simulink model "L4_SIM"  (R2018a)
settings: Solver=ode1  StartTime=0.0  StopTime=60  FixedStep=GLB_FIXED_STEP_SIZE_CPV  RelTol=1e-3  EnableMultiTasking=on
undefined symbols (not defined in the file or in its folder): Cf, Chassis, Cr, CYCLE_ACC1_2A__AdaptiveCruiseCtrlMode, CYCLE_ACC1_2A__AdaptiveCruiseCtrlSetSpeed, CYCLE_CCVS1_00__CruiseCtrlSetSpeed, CYCLE_CCVS1_00__WheelBasedVehicleSpeed, CYCLE_EEC1_00__EngSpeed, CYCLE_ETC1_00__TransDrivelineEngaged, CYCLE_ETC2_00__TransActualGearRatio, CYCLE_ETC7_03__TransMode1Indicator, CYCLE_GPS_Latitude, CYCLE_GPS_Longitude, CYCLE_LFE1_00__EngFuelRate, CYCLE_Net_Engine_Percent_Torque, CYCLE_SSI2_03__PitchAngleExRange, CYCLE_TIME, CYCLE_UTM_Origin_X, CYCLE_UTM_Origin_Y, CYCLE_Vehicle_Distance, DiscIntNeverNeededParam, ENUM_J1939_PCC_STATE_T, ENUM_J1939_SWITCH_T, ENUM_STEERING_WHEEL_ANGLE_SENSOR_TYPE_T, GLB_FIXED_STEP_SIZE_CPV, GLB_TRANS_LOSS_TRQ_GEAR_STEP_MPV, GLB_TRANS_LOSS_TRQ_SPD_STEP_MPV, GLB_TRANS_LOSS_TRQ_TABLE_DATA_MPV, GLB_TRANS_LOSS_TRQ_TRQ_STEP_MPV, GLB_VEHICLE_CONFIG_ACCEL_PED_GATEWAY_APV, heading_0, Iz, L4_Controller, lf, lr, position_0, ptc_matlab_lib, STEERCTRL_10ms, SUB_ECU_L4_MABX, SUB_L4_Task_10ms, SUB_L4_Task_10ms_SUB_STEERCTRL, SUB_PLANT_Chassis, Task_10ms, Vx_0
libraries: EmE_MBD_Blockset x81, PTC_MBDS_LIB x71, simulink x38, simulink_extras x1, SUB_L4_Task_10000ms x1, SUB_L4_Task_1000ms x1, SUB_L4_Task_100ms x1, SUB_L4_Task_10ms_SUB_APTC x1, SUB_L4_Task_10ms_SUB_BRKPEDARB x1, SUB_L4_Task_10ms_SUB_FAULT_MANAGER x1, SUB_L4_Task_10ms_SUB_STATE_CONTROL x1, simulink_need_slupdate x1
(part 4 of 6)

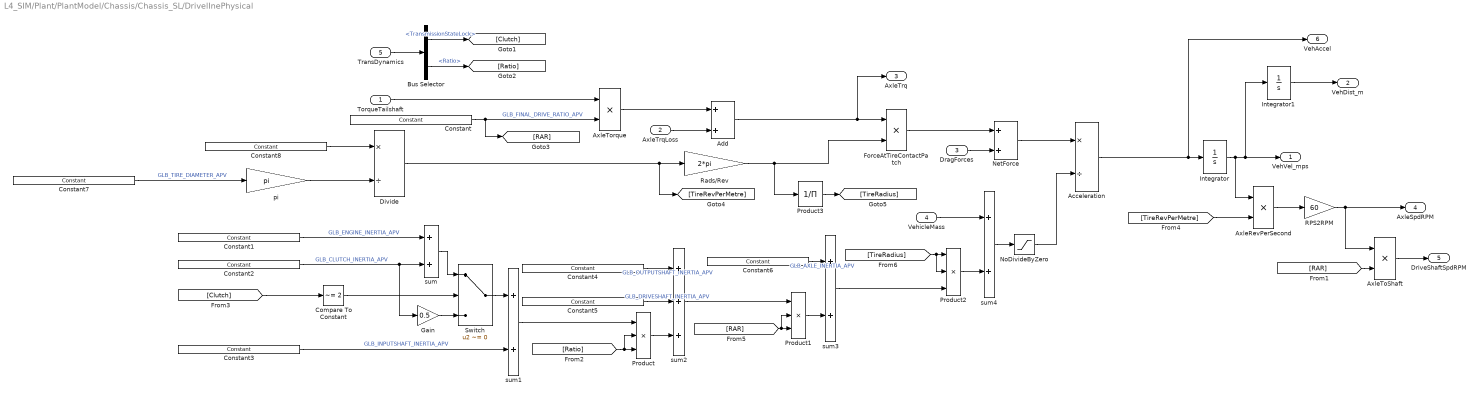
== system L4_SIM/Plant/PlantModel/Chassis/Chassis_SL/DrivelInePhysical ==
  TorqueTailshaft : Inport
  AxleTrqLoss : Inport  Port=2
  DragForces : Inport  Port=3
  VehicleMass : Inport  Port=4
  TransDynamics : Inport  Port=5
  Acceleration : Product  Inputs=*/
  Add : Sum
  AxleRevPerSecond : Product
  AxleToShaft : Product
  AxleTorque : Product
  Bus Selector : BusSelector  OutputSignals=MainClutch_bus.TransmissionStateLock,Gears_bus.Ratio
  Compare To Constant : simulink/Logic and Bit Operations/Compare To Constant  relop=~=  const=2  OutDataTypeStr=boolean
  Constant : PTC_MBDS_LIB/Extras/Sources/Constant  Value2=GLB_FINAL_DRIVE_RATIO_APV  PTC_MBDS_BlockVersion=5.41  PTC_BlockType=PTC_MBDS_Constant
      settings: SourceProductName=PACCAR Technical Center MBDS Library
      settings: AttributesFormatString=|
      | Value: 2.79
      | Unit: '1'
  Constant1 : PTC_MBDS_LIB/Extras/Sources/Constant  Value2=GLB_ENGINE_INERTIA_APV  PTC_MBDS_BlockVersion=5.41  PTC_BlockType=PTC_MBDS_Constant
      settings: SourceProductName=PACCAR Technical Center MBDS Library
      settings: AttributesFormatString=|
      | Value: 3.7109375
      | Unit: 'kg*m^2'
  Constant2 : PTC_MBDS_LIB/Extras/Sources/Constant  Value2=GLB_CLUTCH_INERTIA_APV  PTC_MBDS_BlockVersion=5.41  PTC_BlockType=PTC_MBDS_Constant
      settings: SourceProductName=PACCAR Technical Center MBDS Library
      settings: AttributesFormatString=|
      | Value: 0.115966796875
      | Unit: 'kg*m^2'
  Constant3 : PTC_MBDS_LIB/Extras/Sources/Constant  Value2=GLB_INPUTSHAFT_INERTIA_APV  PTC_MBDS_BlockVersion=5.41  PTC_BlockType=PTC_MBDS_Constant
      settings: SourceProductName=PACCAR Technical Center MBDS Library
      settings: AttributesFormatString=|
      | Value: 0.015
      | Unit: 'kg*m^2'
  Constant4 : PTC_MBDS_LIB/Extras/Sources/Constant  Value2=GLB_OUTPUTSHAFT_INERTIA_APV  PTC_MBDS_BlockVersion=5.41  PTC_BlockType=PTC_MBDS_Constant
      settings: SourceProductName=PACCAR Technical Center MBDS Library
      settings: AttributesFormatString=|
      | Value: 0.03
      | Unit: 'kg*m^2'
  Constant5 : PTC_MBDS_LIB/Extras/Sources/Constant  Value2=GLB_DRIVESHAFT_INERTIA_APV  PTC_MBDS_BlockVersion=5.41  PTC_BlockType=PTC_MBDS_Constant
      settings: SourceProductName=PACCAR Technical Center MBDS Library
      settings: AttributesFormatString=|
      | Value: 0.001
      | Unit: 'kg*m^2'
  Constant6 : PTC_MBDS_LIB/Extras/Sources/Constant  Value2=GLB_AXLE_INERTIA_APV  PTC_MBDS_BlockVersion=5.41  PTC_BlockType=PTC_MBDS_Constant
      settings: SourceProductName=PACCAR Technical Center MBDS Library
      settings: AttributesFormatString=|
      | Value: 0.10000000149
      | Unit: 'kg*m^2'
  Constant7 : PTC_MBDS_LIB/Extras/Sources/Constant  Value2=GLB_TIRE_DIAMETER_APV  PTC_MBDS_BlockVersion=5.41  PTC_BlockType=PTC_MBDS_Constant
      settings: SourceProductName=PACCAR Technical Center MBDS Library
      settings: AttributesFormatString=|
      | Value: 1
      | Unit: 'm'
  Constant8 : PTC_MBDS_LIB/Extras/Sources/Constant  Value2=1  PTC_MBDS_BlockVersion=5.41  PTC_BlockType=PTC_MBDS_Constant
      settings: SourceProductName=PACCAR Technical Center MBDS Library
  Divide : Product  Inputs=*/  OutDataTypeStr=Inherit: Inherit via back propagation  SaturateOnIntegerOverflow=on  InputSameDT=on
      settings: AttributesFormatString=Saturate: %<SaturateOnIntegerOverflow>
  ForceAtTireContactPatch : Product
  Gain : Gain  Gain=0.5
  Integrator : Integrator  InitialCondition=Vx_0  LimitOutput=on  UpperSaturationLimit=1000  LowerSaturationLimit=0
  Integrator1 : Integrator  LimitOutput=on  LowerSaturationLimit=0
  NetForce : Sum
  NoDivideByZero : Saturate  UpperLimit=inf  LowerLimit=1
  Product : Product  Inputs=3
  Product1 : Product  Inputs=3
  Product2 : Product  Inputs=3
  Product3 : Product  Inputs=/
  RPS2RPM : Gain  Gain=60
  Rads/Rev : Gain  Gain=2*pi
  Switch : Switch  Criteria=u2 ~= 0
  pi : Gain  Gain=pi
  sum{,1,3..4} (4 alike) : Sum
  sum2 : Sum  Inputs=3
  VehVel_mps : Outport
  VehDist_m : Outport  Port=2
  AxleTrq : Outport  Port=3
  AxleSpdRPM : Outport  Port=4
  DriveShaftSpdRPM : Outport  Port=5
  VehAccel : Outport  Port=6
  wires:
  Constant8/1 -> Divide/1
  pi/1 -> Divide/2
  Constant7/1 -> pi/1  "GLB_TIRE_DIAMETER_APV"
  VehicleMass/1 -> sum4/1
  Product3/1 -> [TireRadius]
  [TireRadius] -> Product2/1, Product2/2
  sum3/1 -> Product2/3
  sum4/1 -> NoDivideByZero/1
  Product2/1 -> sum4/2
  Product1/1 -> sum3/2
  Constant6/1 -> sum3/1  "GLB_AXLE_INERTIA_APV"
  sum2/1 -> Product1/1
  [RAR] -> Product1/3, Product1/2
  Constant4/1 -> sum2/1  "GLB_OUTPUTSHAFT_INERTIA_APV"
  Constant5/1 -> sum2/2  "GLB_DRIVESHAFT_INERTIA_APV"
  Product/1 -> sum2/3
  sum1/1 -> Product/1
  [Ratio] -> Product/3, Product/2
  Switch/1 -> sum1/1
  Constant3/1 -> sum1/2  "GLB_INPUTSHAFT_INERTIA_APV"
  [RAR] -> AxleToShaft/2
  [TireRevPerMetre] -> AxleRevPerSecond/2
  Bus Selector/2 -> [Ratio]  "<Ratio>"
  Bus Selector/1 -> [Clutch]  "<TransmissionStateLock>"
  sum/1 -> Switch/1
  Gain/1 -> Switch/3
  Constant2/1 -> sum/2, Gain/1  "GLB_CLUTCH_INERTIA_APV"
  Constant1/1 -> sum/1  "GLB_ENGINE_INERTIA_APV"
  Compare To Constant/1 -> Switch/2
  [Clutch] -> Compare To Constant/1
  TransDynamics/1 -> Bus Selector/1
  AxleToShaft/1 -> DriveShaftSpdRPM/1
  RPS2RPM/1 -> AxleSpdRPM/1, AxleToShaft/1
  AxleRevPerSecond/1 -> RPS2RPM/1
  Integrator1/1 -> VehDist_m/1
  Integrator/1 -> VehVel_mps/1, Integrator1/1, AxleRevPerSecond/1
  Acceleration/1 -> Integrator/1, VehAccel/1
  NoDivideByZero/1 -> Acceleration/2
  NetForce/1 -> Acceleration/1
  DragForces/1 -> NetForce/2
  ForceAtTireContactPatch/1 -> NetForce/1
  Add/1 -> ForceAtTireContactPatch/1, AxleTrq/1
  AxleTrqLoss/1 -> Add/2
  Rads/Rev/1 -> ForceAtTireContactPatch/2, Product3/1
  Divide/1 -> Rads/Rev/1, [TireRevPerMetre]
  AxleTorque/1 -> Add/1
  Constant/1 -> AxleTorque/2, [RAR]  "GLB_FINAL_DRIVE_RATIO_APV"
  TorqueTailshaft/1 -> AxleTorque/1

== system L4_SIM/Plant/PlantModel/Chassis/Chassis_SL/Transmission Simple ModeNo SDL ==
  MotorTorqueRequest : Inport
  MainClutchAct : Inport  Port=2
  Gear_No : Inport  Port=3
  Neutral : Inport  Port=4
  EngTrqIn : Inport  Port=5
  EngSpd : Inport  Port=6
  TailShaftSpeed : Inport  Port=7
  Bus Creator : BusCreator  Inputs=3
  Gears : Subsystem
  Main Clutch : Subsystem
  Terminator : Terminator
      settings: InitFcn=|
      | try
      |    MBDS_BlockCallback('Update', gcb);
      | end
  Transmission Dynamics : Outport
  TrqToEng : Outport  Port=2
  ClutchState : Outport  Port=3
  EngSpdClutchClosed : Outport  Port=4
  TransTrqOut : Outport  Port=5
  wires:
  [CommandNeutral] -> Terminator/1
  TailShaftSpeed/1 -> Gears/3(SpdOut)
  Gears/3(TrqOut) -> TransTrqOut/1
  Main Clutch/2(TrqToEngine) -> TrqToEng/1
  Main Clutch/4(ClutchState) -> ClutchState/1
  EngTrqIn/1 -> Main Clutch/2(InputTorque)
  Gears/2(SpdIn) -> EngSpdClutchClosed/1, Main Clutch/3(TransSpd)
  EngSpd/1 -> Main Clutch/4(EngSpd)
  Neutral/1 -> [CommandNeutral]
  MainClutchAct/1 -> Main Clutch/1(Main Clutch Actuator)
  Main Clutch/3(TrqToTransmission) -> Gears/2(TrqIn), [Input_Shft_Trq]
  Gears/1(Gears_o) -> [Gears_O]
  Gear_No/1 -> [NewGear]
  [Gears_O] -> Bus Creator/2  "Gears_bus"
  [MainClutch_O] -> Bus Creator/1  "MainClutch_bus"
  Main Clutch/1(Main Clutch O) -> [MainClutch_O]
  Bus Creator/1 -> Transmission Dynamics/1
  [NewGear] -> Gears/1(Gear)
  [Input_Shft_Trq] -> Bus Creator/3  "s_Input_Shft_Trq"
  MotorTorqueRequest/1 -> Gears/4(MotorTorqueRequest)

== system L4_SIM/Controllers/Operator/Subsystem/SpdControlBrake/SpdControlBrake/PID ==
  Init : Inport
  Reset_Integral : Inport  Port=2
  SP : Inport  Port=3
  FB : Inport  Port=4
  K : Inport  Port=5
  Ti : Inport  Port=6
  Td : Inport  Port=7
  Ts : Inport  Port=8
  Sat_state : Inport  Port=9
  Add : Sum  Inputs=+-
  Add1 : Sum  Inputs=+++
  Add2 : Sum
  Add3 : Sum  Inputs=+-
  AntiWindup : Subsystem
  Divide : Product  Inputs=*/
  Divide1 : Product  Inputs=**/
  Product : Product  RndMeth=Zero
  Product1 : Product  RndMeth=Zero
  Switch : Switch  Criteria=u2 ~= 0
  Unit Delay : UnitDelay  SampleTime=-1
  Unit Delay1 : UnitDelay  SampleTime=-1
  Out1 : Outport
  P_Out : Outport  Port=2
  I_Out : Outport  Port=3
  D_Out1 : Outport  Port=4
  wires:
  AntiWindup/1(I_update_clp) -> Add2/1
  Add2/1 -> Switch/3
  Unit Delay/1 -> I_Out/1, Add1/2, Add2/2
  Switch/1 -> Unit Delay/1
  Td/1 -> Divide1/1
  [KpError] -> Divide1/2
  Sat_state/1 -> AntiWindup/2(Sat_state)
  Product1/1 -> AntiWindup/1(I_update)
  Reset_Integral/1 -> Switch/2
  Init/1 -> Switch/1
  SP/1 -> Add/1
  FB/1 -> Add/2
  Add/1 -> Product/1
  K/1 -> Product/2
  Product/1 -> Product1/1, Add1/1, P_Out/1, [KpError]
  Ts/1 -> Divide1/3, Divide/1
  Ti/1 -> Divide/2
  Divide/1 -> Product1/2
  Add1/1 -> Out1/1
  Divide1/1 -> Add3/1, Unit Delay1/1
  Unit Delay1/1 -> Add3/2
  Add3/1 -> Add1/3, D_Out1/1

== system L4_SIM/Controllers/Operator/Subsystem/SpdControlTraction/SpdControlTraction/PID ==
  Init : Inport
  Reset_Integral : Inport  Port=2
  SP : Inport  Port=3
  FB : Inport  Port=4
  K : Inport  Port=5
  Ti : Inport  Port=6
  Td : Inport  Port=7
  Ts : Inport  Port=8
  Sat_state : Inport  Port=9
  Add : Sum  Inputs=+-
  Add1 : Sum  Inputs=+++
  Add2 : Sum
  Add3 : Sum  Inputs=+-
  AntiWindup : Subsystem
  Divide : Product  Inputs=*/
  Divide1 : Product  Inputs=**/
  Product : Product  RndMeth=Zero
  Product1 : Product  RndMeth=Zero
  Switch : Switch  Criteria=u2 ~= 0
  Unit Delay : UnitDelay  SampleTime=-1
  Unit Delay1 : UnitDelay  SampleTime=-1
  Out1 : Outport
  P_Out : Outport  Port=2
  I_Out : Outport  Port=3
  D_Out1 : Outport  Port=4
  wires:
  Sat_state/1 -> AntiWindup/2(Sat_state)
  Product1/1 -> AntiWindup/1(I_update)
  AntiWindup/1(I_update_clp) -> Add2/1
  Reset_Integral/1 -> Switch/2
  Init/1 -> Switch/1
  SP/1 -> Add/1
  FB/1 -> Add/2
  Add/1 -> Product/1
  K/1 -> Product/2
  Product/1 -> Product1/1, Add1/1, P_Out/1, [KpError]
  Ts/1 -> Divide1/3, Divide/1
  Ti/1 -> Divide/2
  Divide/1 -> Product1/2
  Unit Delay/1 -> Add2/2
  Switch/1 -> Unit Delay/1
  Add2/1 -> Add1/2, I_Out/1, Switch/3
  Add1/1 -> Out1/1
  Td/1 -> Divide1/1
  [KpError] -> Divide1/2
  Divide1/1 -> Add3/1, Unit Delay1/1
  Unit Delay1/1 -> Add3/2
  Add3/1 -> Add1/3, D_Out1/1

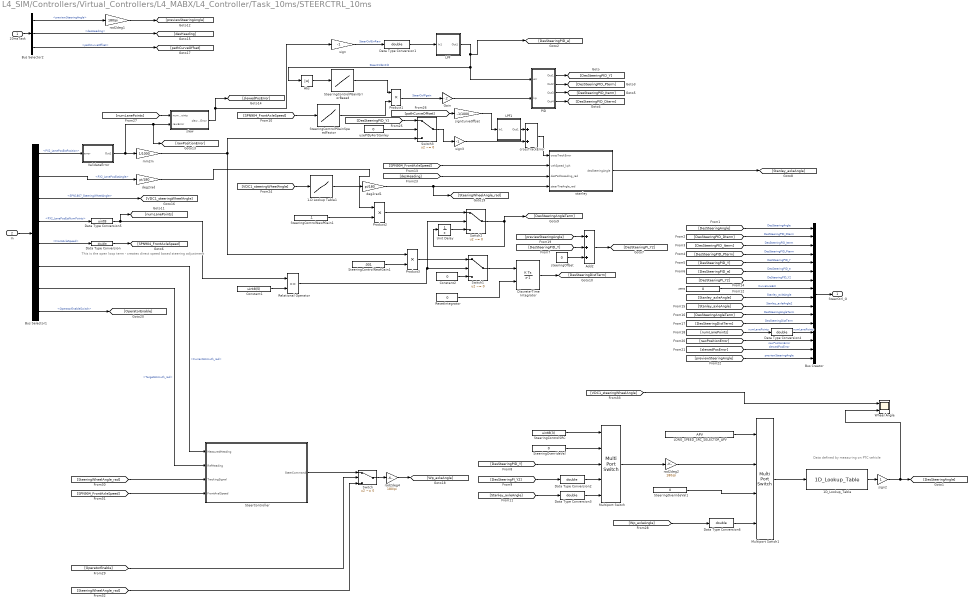
== system L4_SIM/Controllers/Virtual_Controllers/L4_MABX/L4_Controller/Task_10ms/STEERCTRL_10ms ==
  note: Data defined by measuring on PTC vehicle
  note: This is the open loop term - creates direct speed based steering adjustment
  20msTask : Inport
  In : Inport  Port=2
  1-D Lookup Table1 : Lookup_n-D  NumberOfTableDimensions=1  BreakpointsForDimension1=|  Table=|  InternalRulePriority=Speed  RndMeth=Simplest  InputSameDT=on
      BreakpointsForDimension1=|
      | [-800
      | -700
      | -600
      | -500
      | -400
      | -300
      | -200
      | -100
      | 0
      | 100
      | 200
      | 300
      | 400
      | 500
      | 600
      | 700
      | 800
      | ]
      Table=|
      | [-46
      | -39.5
      | -33.5
      | -27
      | -21.5
      | -16
      | -10
      | -4.5
      | 0
      | 5.5
      | 11
      | 16
      | 21.5
      | 26
      | 31
      | 33
      | 33
      | ]
  1D_Lookup_Table : PTC_MBDS_LIB/Extras/Lookup Tables/1D_Lookup_Table  ParameterObjectName=STEERCTRL_WHEEL_ANGLE_DATA_MPV  InterpolationMethod=Linear  PTC_MBDS_BlockVersion=5.41  PTC_BlockType=PTC_MBDS_1D_Lookup_Table
      settings: SourceProductName=PACCAR Technical Center MBDS Library
      settings: AttributesFormatString=|
      | X Axis: STEERCTRL_WHEEL_ANGLE_STEP_MPV (deg)
      | Y Axis: STEERCTRL_WHEEL_ANGLE_DATA_MPV (deg)
      | Interpolation Method: Linear
  Abs : Abs
  Add2 : Sum  Inputs=+++
  Bus Creator : BusCreator  Inputs=16
  Bus Selector1 : BusSelector  OutputSignals=CAN.PX2_Lane.LanePosEst.PX2_LanePosEstPosition,CAN.PX2_Lane.LanePosEst.PX2_LanePosEstAngle,CAN.VDC2_0B.SPN1807_SteeringWheelAngle,CAN.PX2_Lane.LanePosEst.PX2_LanePosEstNumPoints,CAN.EBC2_0B.FrontAxleSpeed,PIC_Bus.CurrentAzimuth_rad,PIC_Bus.TargetAzimuth_rad,DIO_Bus.OperatorEnableSwitch
  Bus Selector2 : BusSelector  OutputSignals=mapping.previewSteeringAngle,mapping.desHeading,mapping.pathCurveOffset
  Constant1 : Constant  Value=uint8(5)
  Constant2 : Constant  Value=0
  Data Type Conversion{,1..4,6} (6 alike) : DataTypeConversion  OutDataTypeStr=double
  Data Type Conversion5 : DataTypeConversion  OutDataTypeStr=uint8
  Discrete-Time Integrator : DiscreteIntegrator  ExternalReset=level  SampleTime=.01  LimitOutput=on  UpperSaturationLimit=1000  LowerSaturationLimit=-1000  ICPrevOutput=DiscIntNeverNeededParam  ICPrevScaledInput=DiscIntNeverNeededParam
  Gain : Gain  Gain=-.2
  LONG_SPEED_SRC_SELECTOR_APV : EmE_MBD_Blockset/Sources/APV  conval=LONG_SPEED_SRC_SELECTOR_APV
      settings: SourceProductName=PACCAR EmE MBD Blockset
  LPF : Subsystem
  LPF1 : Subsystem
  Multiport Switch : MultiPortSwitch  DataPortOrder=Zero-based contiguous  Inputs=4  zeroidx=on
  Multiport Switch1 : MultiPortSwitch  DataPortOrder=Specify indices  DataPortIndices={ENUM_LONG_SPEED_DEMAND_SOURCE_T.GPS_PATH,ENUM_LONG_SPEED_DEMAND_SOURCE_T.OVERRIDE,ENUM_LONG_SPEED_DEMAND_SOURCE_T.RW_WAYPOINTS}  DiagnosticForDefault=None
  PID : Subsystem
  Product1 : Product
  Product2 : Product
  Product3 : Product
  Relational Operator : RelationalOperator  OutDataTypeStr=boolean  RndMeth=Nearest
  ResetIntegrator : Constant  Value=0
  SteerController : Subsystem
  SteeringControlNewIGain1 : Constant  Value=.001
  SteeringControlNewPGain1 : Constant  Value=.1
  SteeringControlPGainErrorBased : Lookup_n-D  NumberOfTableDimensions=1  BreakpointsForDimension1=[0 .005 .01 .02 .035 .05 .1 .2 .3 .5]  Table=[100 250 300 400 500 500 400 400 400 200]  InternalRulePriority=Speed  RndMeth=Simplest  InputSameDT=on
  SteeringControlPGainSpeedFactor : Lookup_n-D  NumberOfTableDimensions=1  BreakpointsForDimension1=[10 20 30 40 50 60 70 80 90]  Table=[.5 .5 .43 .38 .3 .2 .2 .2 .2]  InternalRulePriority=Speed  RndMeth=Simplest  InputSameDT=on
  SteeringControlSRC : Constant  Value=uint8(3)
  SteeringOverrideVal : Constant  Value=0
  SteeringOverrideVal1 : Constant  Value=0
  Switch{,1..3} (4 alike) : Switch  Criteria=u2 ~= 0
  Unit Delay : UnitDelay  SampleTime=-1
  ValidateError : Subsystem
  Wheel Angle : Scope  NumInputPorts=2
  crossTrackError : Sum
  deg2rad : Gain  Gain=pi/180
  deg2rad1 : Gain  Gain=pi/180
  mm2m : Gain  Gain=1/1000  OutDataTypeStr=double
  rad2deg1 : Gain  Gain=180/pi
  rad2deg2 : Gain  Gain=180/pi
  rad2deg4 : Gain  Gain=180/pi
  sign : Gain  Gain=-1
  sign2 : Gain
  sign3 : Gain  Gain=-1
  signCurveOffset : Gain  Gain=-1/1000
  slew : Subsystem
  stanley : Subsystem
  steeringOffset : Constant  Value=0
  usePIDyForStanley : Constant  Value=0
  zero : Constant  Value=0
  SteerCtrl_O : Outport
  wires:
  SteeringOverrideVal/1 -> Multiport Switch/2
  [SPN904_FrontAxleSpeed] -> stanley/2(vehSpeed_kph)
  Switch/1 -> rad2deg4/1
  Bus Selector1/8 -> [OperatorEnable]  "<OperatorEnableSwitch>"
  [previewSteeringAngle] -> Bus Creator/16  "previewSteeringAngle"
  LPF1/1(Out1) -> crossTrackError/1
  Bus Selector1/5 -> Data Type Conversion/1  "<FrontAxleSpeed>"
  SteeringControlNewIGain1/1 -> Product3/2
  Bus Selector2/2 -> [desHeading]  "<desHeading>"
  Bus Selector1/6 -> SteerController/1(MeasuredHeading)  "<CurrentAzimuth_rad>"
  usePIDyForStanley/1 -> Switch3/2
  [SteeringWheelAngle_rad] -> Switch/3
  rad2deg2/1 -> Multiport Switch1/2
  ValidateError/1(Out1) -> [rawPositionError], slew/2(rawError), mm2m/1
  [SteeringWheelAngle_rad] -> SteerController/3(TrackingSignal)
  Bus Creator/1 -> SteerCtrl_O/1
  [DesSteeringAngle] -> Bus Creator/1  "DesSteeringAngle"
  [desHeading] -> stanley/3(desPathHeading_rad)
  [SPN904_FrontAxleSpeed] -> SteerController/4(FrontAxelSpeed)
  1D_Lookup_Table/1 -> sign2/1
  SteeringControlPGainSpeedFactor/1 -> Product1/2
  Data Type Conversion5/1 -> Relational Operator/1, [numLanePoints]
  [previewSteeringAngle] -> Add2/1
  sign3/1 -> crossTrackError/2
  PID/2(Out2) -> [DesSteeringPID_Pterm]
  Data Type Conversion2/1 -> Multiport Switch/4
  Bus Selector2/3 -> [pathCurveOffset]  "<pathCurveOffset>"
  Multiport Switch/1 -> rad2deg2/1
  slew/1(slewedError) -> [slewedPosError], sign/1
  [rawPositionError] -> Bus Creator/14  "rawPositionError"
  SteeringOverrideVal1/1 -> Multiport Switch1/3
  sign2/1 -> Wheel Angle/2, [DesSteeringAngle]
  Bus Selector1/7 -> SteerController/2(RefHeading)  "<TargetAzimuth_rad>"
  SteerController/1(SteerCommand) -> Switch/1
  Bus Selector1/3 -> [VDC1_steeringWheelAngle]  "<SPN1807_SteeringWheelAngle>"
  Data Type Conversion6/1 -> Multiport Switch1/4
  Multiport Switch1/1 -> 1D_Lookup_Table/1
  [slewedPosError] -> Bus Creator/15  "slewedPosError"
  Switch3/1 -> sign3/1
  crossTrackError/1 -> stanley/1(crossTrackError)
  [DesSteeringPID_Y] -> Multiport Switch/3
  [SPN904_FrontAxleSpeed] -> SteeringControlPGainSpeedFactor/1
  signCurveOffset/1 -> LPF1/1(In1)
  stanley/1(desSteeringAngle) -> [Stanley_axleAngle]
  [numLanePoints] -> slew/1(numLanePoints)
  Data Type Conversion1/1 -> LPF/1(In1)
  Bus Selector1/1 -> ValidateError/1(error)  "<PX2_LanePosEstPosition>"
  [numLanePoints] -> Data Type Conversion4/1  "numLanePoints"
  steeringOffset/1 -> Add2/3
  [DesSteeringPID_Y] -> Switch3/1
  rad2deg1/1 -> [previewSteeringAngle]
  PID/4(Out4) -> [DesSteeringPID_Dterm]
  PID/1(Out1) -> [DesSteeringPID_Y]
  In/1 -> Bus Selector1/1
  Abs/1 -> SteeringControlPGainErrorBased/1
  [DesSteeringPID_Y] -> Add2/2
  Constant2/1 -> Switch1/3
  LONG_SPEED_SRC_SELECTOR_APV/1 -> Multiport Switch1/1
  Switch1/1 -> Discrete-Time Integrator/1
  [DesSteeringDistTerm] -> Bus Creator/12  "DesSteeringDistTerm"
  [DesSteeringPID_Dterm] -> Bus Creator/2  "DesSteeringPID_Dterm"
  Bus Selector2/1 -> rad2deg1/1  "<previewSteeringAngle>"
  [OperatorEnable] -> Switch/2
  [DesSteeringPI_Y2] -> Bus Creator/7  "DeSteeringPID_Y2"
  [Stanley_axleAngle] -> Bus Creator/9  "Stanley_axleAngle"
  [Stanley_axleAngle] -> Data Type Conversion3/1
  Discrete-Time Integrator/1 -> [DesSteeringDistTerm]
  SteeringControlSRC/1 -> Multiport Switch/1
  Product2/1 -> Switch2/1
  [pathCurveOffset] -> signCurveOffset/1
  [DesSteeringPI_Y2] -> Data Type Conversion2/1
  [VDC1_steeringWheelAngle] -> Wheel Angle/1
  Data Type Conversion3/1 -> Multiport Switch/5
  Data Type Conversion4/1 -> Bus Creator/13  "numLanePoints"
  deg2rad1/1 -> stanley/4(steerTireAngle_rad), [SteeringWheelAngle_rad]
  [DesSteeringAngleTerm] -> Bus Creator/11  "DesSteeringAngleTerm"
  zero/1 -> Bus Creator/8  "CurvatureEst"
  Constant1/1 -> Relational Operator/2
  ResetIntegrator/1 -> Discrete-Time Integrator/2
  Gain/1 -> PID/2(kp)
  Product1/1 -> Gain/1  "SteerCtrlPgain"
  SteeringControlNewPGain1/1 -> Product2/2
  rad2deg4/1 -> [Wp_axleAngle]
  Add2/1 -> [DesSteeringPI_Y2]
  Data Type Conversion/1 -> [SPN904_FrontAxleSpeed]
  Unit Delay/1 -> Switch2/3
  [DesSteeringPID_Pterm] -> Bus Creator/4  "DesSteeringPID_Pterm"
  [DesSteeringPID_e] -> Bus Creator/6  "DesSteeringPID_e"
  [DesSteeringPID_Y] -> Bus Creator/5  "DesSteeringPID_Y"
  Bus Selector1/4 -> Data Type Conversion5/1  "<PX2_LanePosEstNumPoints>"
  [Wp_axleAngle] -> Data Type Conversion6/1
  Product3/1 -> Switch1/1
  [VDC1_steeringWheelAngle] -> 1-D Lookup Table1/1
  [Stanley_axleAngle] -> Bus Creator/10  "Stanley_axleAngle2"
  deg2rad/1 -> Product2/1
  PID/3(Out3) -> [DesSteeringPID_Iterm]
  SteeringControlPGainErrorBased/1 -> Product1/1
  LPF/1(Out1) -> [DesSteeringPID_e], PID/1(err), Abs/1  "SteerCtrlErrFilt"
  mm2m/1 -> Switch3/3, Product3/1
  [DesSteeringPID_Iterm] -> Bus Creator/3  "DesSteeringPID_Iterm"
  Switch2/1 -> [DesSteeringAngleTerm], Unit Delay/1
  20msTask/1 -> Bus Selector2/1
  Relational Operator/1 -> Switch2/2, Switch1/2
  sign/1 -> Data Type Conversion1/1  "SteerCtrlErrRaw"
  1-D Lookup Table1/1 -> deg2rad1/1
  Bus Selector1/2 -> deg2rad/1  "<PX2_LanePosEstAngle>"

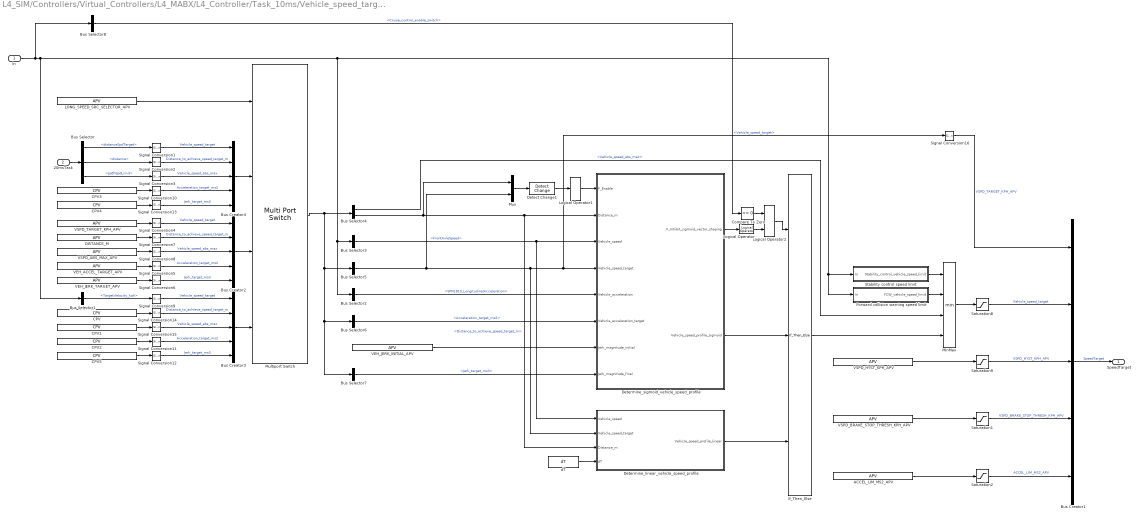
== system L4_SIM/Controllers/Virtual_Controllers/L4_MABX/L4_Controller/Task_10ms/Vehicle_speed_target ==
  In : Inport
  20msTask : Inport  Port=2
  ACCEL_LIM_MS2_APV : EmE_MBD_Blockset/Sources/APV  conval=-5
      settings: SourceProductName=PACCAR EmE MBD Blockset
  Bus Creator{1..4} (4 alike) : BusCreator  Inputs=5
  Bus Selector : BusSelector  OutputSignals=mapping.distanceSpdTarget,mapping.distance,mapping.pathSpdLimit
  Bus Selector1 : BusSelector  OutputSignals=PIC_Bus.TargetVelocity_kph
  Bus Selector2 : BusSelector  OutputSignals=CAN.VDC2_0B.SPN1810_LongitudinalAcceleration
  Bus Selector3 : BusSelector  OutputSignals=CAN.EBC2_0B.FrontAxleSpeed
  Bus Selector4 : BusSelector  OutputSignals=Vehicle_speed_abs_max,Distance_to_achieve_speed_target_m
  Bus Selector5 : BusSelector  OutputSignals=Vehicle_speed_target
  Bus Selector6 : BusSelector  OutputSignals=Acceleration_target_ms2
  Bus Selector7 : BusSelector  OutputSignals=Jerk_target_ms3
  Bus Selector8 : BusSelector  OutputSignals=CAN.CCVS_31.Cruise_control_enable_switch
  CPV{,2..4} (4 alike) : EmE_MBD_Blockset/Sources/CPV  conval=0
      settings: SourceProductName=PACCAR EmE MBD Blockset
  CPV1 : EmE_MBD_Blockset/Sources/CPV  conval=255
      settings: SourceProductName=PACCAR EmE MBD Blockset
  CPV5 : EmE_MBD_Blockset/Sources/CPV  conval=0.5
      settings: SourceProductName=PACCAR EmE MBD Blockset
  Compare To Zero : simulink/Logic and Bit Operations/Compare To Zero  relop===  OutDataTypeStr=boolean
  DISTANCE_M : EmE_MBD_Blockset/Sources/APV  conval=200
      settings: SourceProductName=PACCAR EmE MBD Blockset
  Detect Change1 : simulink/Logic and Bit Operations/Detect Change  vinit=0  InputProcessing=Inherited  OutDataTypeStr=boolean
      settings: AttributesFormatString=IC: %<vinit>
  Determine_linear_vehicle_speed_profile : Subsystem
  Determine_sigmoid_vehicle_speed_profile : Subsystem
  Forward collision warning speed limit : Subsystem
  If_Then_Else : EmE_MBD_Blockset/Signal Routing/If_Then_Else
      settings: SourceProductName=PACCAR EmE MBD Blockset
  LONG_SPEED_SRC_SELECTOR_APV : EmE_MBD_Blockset/Sources/APV  conval=LONG_SPEED_SRC_SELECTOR_APV
      settings: SourceProductName=PACCAR EmE MBD Blockset
  Logical Operator : EmE_MBD_Blockset/Logic and Bit Operations/Logical Operator  Operator=NOT  Inputs=2
      settings: SourceProductName=PACCAR EmE MBD Blockset
  Logical Operator1 : EmE_MBD_Blockset/Logic and Bit Operations/Logical Operator  Operator=OR  Inputs=1
      settings: SourceProductName=PACCAR EmE MBD Blockset
  Logical Operator2 : EmE_MBD_Blockset/Logic and Bit Operations/Logical Operator  Operator=AND  Inputs=2
      settings: SourceProductName=PACCAR EmE MBD Blockset
  MinMax : MinMax  Inputs=4  InputSameDT=on
  Multiport Switch : MultiPortSwitch  DataPortOrder=Specify indices  DataPortIndices={ENUM_LONG_SPEED_DEMAND_SOURCE_T.GPS_PATH,ENUM_LONG_SPEED_DEMAND_SOURCE_T.OVERRIDE,ENUM_LONG_SPEED_DEMAND_SOURCE_T.RW_WAYPOINTS}  DiagnosticForDefault=None
  Mux : Mux  Inputs=2
  Saturation1 : Saturate  UpperLimit=5  LowerLimit=0
      settings: AttributesFormatString=|
      | Min: %<LowerLimit>
      | Max: %<UpperLimit>
  Saturation2 : Saturate  UpperLimit=15.562  LowerLimit=-15.562
      settings: AttributesFormatString=|
      | Min: %<LowerLimit>
      | Max: %<UpperLimit>
  Saturation8 : Saturate  UpperLimit=100  LowerLimit=0
      settings: AttributesFormatString=|
      | Min: %<LowerLimit>
      | Max: %<UpperLimit>
  Saturation9 : Saturate  UpperLimit=5  LowerLimit=0
      settings: AttributesFormatString=|
      | Min: %<LowerLimit>
      | Max: %<UpperLimit>
  Signal Conversion{1..16} (16 alike) : SignalConversion  OverrideOpt=off
  Stability control speed limit : Subsystem
  VEH_ACCEL_TARGET_APV : EmE_MBD_Blockset/Sources/APV  conval=-0.5
      settings: SourceProductName=PACCAR EmE MBD Blockset
  VEH_JERK_INITIAL_APV : EmE_MBD_Blockset/Sources/APV  conval=0.4
      settings: SourceProductName=PACCAR EmE MBD Blockset
  VEH_JERK_TARGET_APV : EmE_MBD_Blockset/Sources/APV  conval=0.2
      settings: SourceProductName=PACCAR EmE MBD Blockset
  VSPD_ABS_MAX_APV : EmE_MBD_Blockset/Sources/APV  conval=255
      settings: SourceProductName=PACCAR EmE MBD Blockset
  VSPD_BRAKE_STOP_THRESH_KPH_APV : EmE_MBD_Blockset/Sources/APV  conval=2
      settings: SourceProductName=PACCAR EmE MBD Blockset
  VSPD_HYST_KPH_APV : EmE_MBD_Blockset/Sources/APV  conval=1
      settings: SourceProductName=PACCAR EmE MBD Blockset
  VSPD_TARGET_KPH_APV : EmE_MBD_Blockset/Sources/APV  conval=0
      settings: SourceProductName=PACCAR EmE MBD Blockset
  dT : EmE_MBD_Blockset/Sources/dT
      settings: SourceProductName=PACCAR EmE MBD Blockset
  SpeedTarget : Outport
  wires:
  In/1 -> Bus Selector8/1, Bus Selector1/1, Bus Selector2/1, Bus Selector3/1, Stability control speed limit/1(In), Forward collision warning speed limit/1(In)
  VSPD_HYST_KPH_APV/1 -> Saturation9/1
  Saturation8/1 -> Bus Creator1/2  "Vehicle_speed_target"
  Stability control speed limit/1(Stability_control_vehicle_speed_limit) -> MinMax/1
  LONG_SPEED_SRC_SELECTOR_APV/1 -> Multiport Switch/1
  Saturation1/1 -> Bus Creator1/4  "VSPD_BRAKE_STOP_THRESH_KPH_APV"
  MinMax/1 -> Saturation8/1
  VSPD_BRAKE_STOP_THRESH_KPH_APV/1 -> Saturation1/1
  ACCEL_LIM_MS2_APV/1 -> Saturation2/1
  Bus Selector1/1 -> Signal Conversion9/1  "<TargetVelocity_kph>"
  Saturation2/1 -> Bus Creator1/5  "ACCEL_LIM_MS2_APV"
  Saturation9/1 -> Bus Creator1/3  "VSPD_HYST_KPH_APV"
  Bus Creator1/1 -> SpeedTarget/1  "SpeedTarget"
  Determine_linear_vehicle_speed_profile/1(Vehicle_speed_profile_linear) -> If_Then_Else/3
  Determine_sigmoid_vehicle_speed_profile/1(F_Inhibit_sigmoid_vector_shaping) -> Logical Operator/1
  Bus Selector2/1 -> Determine_sigmoid_vehicle_speed_profile/5(Vehicle_acceleration)  "<SPN1810_LongitudinalAcceleration>"
  dT/1 -> Determine_linear_vehicle_speed_profile/4(dT)
  Logical Operator1/1 -> Determine_sigmoid_vehicle_speed_profile/1(F_Enable)
  Bus Selector3/1 -> Determine_sigmoid_vehicle_speed_profile/3(Vehicle_speed), Determine_linear_vehicle_speed_profile/1(Vehicle_speed)  "<FrontAxleSpeed>"
  Bus Selector4/2 -> Determine_sigmoid_vehicle_speed_profile/2(Distance_m), Determine_linear_vehicle_speed_profile/3(Distance_m), Mux/1  "<Distance_to_achieve_speed_target_m>"
  Logical Operator/1 -> Logical Operator2/2
  Bus Selector6/1 -> Determine_sigmoid_vehicle_speed_profile/6(Vehicle_acceleration_target)  "<Acceleration_target_ms2>"
  Bus Selector/2 -> Signal Conversion2/1  "<distance>"
  20msTask/1 -> Bus Selector/1
  If_Then_Else/1 -> MinMax/4
  Bus Creator4/1 -> Multiport Switch/2
  VSPD_TARGET_KPH_APV/1 -> Signal Conversion4/1
  DISTANCE_M/1 -> Signal Conversion7/1
  Bus Selector/1 -> Signal Conversion1/1  "<distanceSpdTarget>"
  Bus Selector/3 -> Signal Conversion3/1  "<pathSpdLimit>"
  VSPD_ABS_MAX_APV/1 -> Signal Conversion8/1
  CPV/1 -> Signal Conversion14/1
  CPV1/1 -> Signal Conversion15/1
  Multiport Switch/1 -> Bus Selector7/1, Bus Selector6/1, Bus Selector5/1, Bus Selector4/1
  Signal Conversion3/1 -> Bus Creator4/3  "Vehicle_speed_abs_max"
  Signal Conversion2/1 -> Bus Creator4/2  "Distance_to_achieve_speed_target_m"
  Signal Conversion1/1 -> Bus Creator4/1  "Vehicle_speed_target"
  Signal Conversion10/1 -> Bus Creator4/4  "Acceleration_target_ms2"
  CPV2/1 -> Signal Conversion11/1
  CPV3/1 -> Signal Conversion10/1
  Bus Selector4/1 -> MinMax/3  "<Vehicle_speed_abs_max>"
  Forward collision warning speed limit/1(FCW_vehicle_speed_limit) -> MinMax/2
  Detect Change1/1 -> Logical Operator1/1
  Mux/1 -> Detect Change1/1
  Bus Selector5/1 -> Determine_linear_vehicle_speed_profile/2(Vehicle_speed_target), Signal Conversion16/1, Determine_sigmoid_vehicle_speed_profile/4(Vehicle_speed_target), Mux/2  "<Vehicle_speed_target>"
  Determine_sigmoid_vehicle_speed_profile/2(Vehicle_speed_profile_sigmoid) -> If_Then_Else/2
  CPV4/1 -> Signal Conversion13/1
  Signal Conversion13/1 -> Bus Creator4/5  "Jerk_target_ms3"
  Signal Conversion6/1 -> Bus Creator2/5  "Jerk_target_ms3"
  Signal Conversion5/1 -> Bus Creator2/4  "Acceleration_target_ms2"
  Signal Conversion4/1 -> Bus Creator2/1  "Vehicle_speed_target"
  Signal Conversion7/1 -> Bus Creator2/2  "Distance_to_achieve_speed_target_m"
  Signal Conversion8/1 -> Bus Creator2/3  "Vehicle_speed_abs_max"
  Bus Creator2/1 -> Multiport Switch/3
  VEH_ACCEL_TARGET_APV/1 -> Signal Conversion5/1
  VEH_JERK_TARGET_APV/1 -> Signal Conversion6/1
  Bus Creator3/1 -> Multiport Switch/4
  Signal Conversion15/1 -> Bus Creator3/3  "Vehicle_speed_abs_max"
  Signal Conversion14/1 -> Bus Creator3/2  "Distance_to_achieve_speed_target_m"
  Signal Conversion9/1 -> Bus Creator3/1  "Vehicle_speed_target"
  Signal Conversion11/1 -> Bus Creator3/4  "Acceleration_target_ms2"
  Signal Conversion12/1 -> Bus Creator3/5  "Jerk_target_ms3"
  CPV5/1 -> Signal Conversion12/1
  Bus Selector7/1 -> Determine_sigmoid_vehicle_speed_profile/8(Jerk_magnitude_final)  "<Jerk_target_ms3>"
  VEH_JERK_INITIAL_APV/1 -> Determine_sigmoid_vehicle_speed_profile/7(Jerk_magnitude_initial)
  Logical Operator2/1 -> If_Then_Else/1
  Bus Selector8/1 -> Compare To Zero/1  "<Cruise_control_enable_switch>"
  Compare To Zero/1 -> Logical Operator2/1
  Signal Conversion16/1 -> Bus Creator1/1  "VSPD_TARGET_KPH_APV"

== system L4_SIM/Plant/PlantModel/Chassis/Chassis_SL/Chassis/Brakes ==
  BrkPress : Inport
  BrakePrimarySupplyPressure_kpa : Inport  Port=2
  WheelSpdRPM : Inport  Port=3
  1-D Lookup Table : Lookup_n-D  NumberOfTableDimensions=1  BreakpointsForDimension1=[0 .1 1 10]  Table=[0 .1 .5 1]  ExtrapMethod=Clip  UseLastTableValue=on  RndMeth=Simplest  InputSameDT=on
  BrakeTorq Table : Lookup_n-D  NumberOfTableDimensions=1  BreakpointsForDimension1=[0:.1:1]  Table=[0 100 500 1000 2000 4000 8000 16000 20000 24000 50000]  RndMeth=Simplest  InputSameDT=on
  Gain : Gain  Gain=10
  NetBrakeTrq : Product  RndMeth=Zero
  Product : Product  RndMeth=Zero
  BrakeTorque : Outport
  BrakeApplicationPressure_kpa : Outport  Port=2
  wires:
  BrakePrimarySupplyPressure_kpa/1 -> Product/1
  Product/1 -> BrakeApplicationPressure_kpa/1
  Gain/1 -> BrakeTorque/1
  NetBrakeTrq/1 -> Gain/1
  1-D Lookup Table/1 -> NetBrakeTrq/2
  BrkPress/1 -> Product/2, BrakeTorq Table/1
  BrakeTorq Table/1 -> NetBrakeTrq/1
  WheelSpdRPM/1 -> 1-D Lookup Table/1

== system L4_SIM/Plant/PlantModel/Chassis/Chassis_SL/Chassis/Rolling Losses1 ==
  Front Axle Load N : Inport
  Drive Axle Load N : Inport  Port=2
  Trailer Axle Load N : Inport  Port=3
  VehSpd(m/s) : Inport  Port=4
  2D_Lookup_Table : PTC_MBDS_LIB/Extras/Lookup Tables/2D_Lookup_Table  ParameterObjectName=GLB_STEER_TIRE_RRVSLOAD_RES_MPV  InterpolationMethod=Linear  PTC_MBDS_BlockVersion=5.41  PTC_BlockType=PTC_MBDS_2D_Lookup_Table
      settings: SourceProductName=PACCAR Technical Center MBDS Library
      settings: AttributesFormatString=|
      | Row Axis: GLB_STEER_TIRE_RRVSLOAD_TREAD_MPV (in/32)
      | Column Axis: GLB_STEER_TIRE_RRVSLOAD_LOAD_MPV (N)
      | Data Axis: GLB_STEER_TIRE_RRVSLOAD_RES_MPV (N)
      | Interpolation Method: Linear
  2D_Lookup_Table1 : PTC_MBDS_LIB/Extras/Lookup Tables/2D_Lookup_Table  ParameterObjectName=GLB_DRIVE_TIRE_RRVSLOAD_RES_MPV  InterpolationMethod=Linear  PTC_MBDS_BlockVersion=5.41  PTC_BlockType=PTC_MBDS_2D_Lookup_Table
      settings: SourceProductName=PACCAR Technical Center MBDS Library
      settings: AttributesFormatString=|
      | Row Axis: GLB_DRIVE_TIRE_RRVSLOAD_TREAD_MPV (in/32)
      | Column Axis: GLB_DRIVE_TIRE_RRVSLOAD_LOAD_MPV (N)
      | Data Axis: GLB_DRIVE_TIRE_RRVSLOAD_RES_MPV (N)
      | Interpolation Method: Linear
  2D_Lookup_Table2 : PTC_MBDS_LIB/Extras/Lookup Tables/2D_Lookup_Table  ParameterObjectName=GLB_TRAILER_TIRE_RRVSLOAD_RES_MPV  InterpolationMethod=Linear  PTC_MBDS_BlockVersion=5.41  PTC_BlockType=PTC_MBDS_2D_Lookup_Table
      settings: SourceProductName=PACCAR Technical Center MBDS Library
      settings: AttributesFormatString=|
      | Row Axis: GLB_TRAILER_TIRE_RRVSLOAD_TREAD_MPV (in/32)
      | Column Axis: GLB_TRAILER_TIRE_RRVSLOAD_LOAD_MPV (N)
      | Data Axis: GLB_TRAILER_TIRE_RRVSLOAD_RES_MPV (N)
      | Interpolation Method: Linear
  Add4 : Sum  Inputs=+++
  Bus Creator : BusCreator  Inputs=5
  Constant : PTC_MBDS_LIB/Extras/Sources/Constant  Value2=GLB_STEER_TREAD_APV  PTC_MBDS_BlockVersion=5.41  PTC_BlockType=PTC_MBDS_Constant
      settings: SourceProductName=PACCAR Technical Center MBDS Library
      settings: AttributesFormatString=|
      | Value: 24
      | Unit: 'in/32'
  Constant1 : PTC_MBDS_LIB/Extras/Sources/Constant  Value2=GLB_NUMBER_OF_FRONT_TIRES_APV  PTC_MBDS_BlockVersion=5.41  PTC_BlockType=PTC_MBDS_Constant
      settings: SourceProductName=PACCAR Technical Center MBDS Library
      settings: AttributesFormatString=|
      | Value: 2
      | Unit: '1'
  Constant2 : PTC_MBDS_LIB/Extras/Sources/Constant  Value2=GLB_DRIVE_TREAD_APV  PTC_MBDS_BlockVersion=5.41  PTC_BlockType=PTC_MBDS_Constant
      settings: SourceProductName=PACCAR Technical Center MBDS Library
      settings: AttributesFormatString=|
      | Value: 24
      | Unit: 'in/32'
  Constant3 : PTC_MBDS_LIB/Extras/Sources/Constant  Value2=GLB_NUMBER_OF_REAR_TIRES_APV  PTC_MBDS_BlockVersion=5.41  PTC_BlockType=PTC_MBDS_Constant
      settings: SourceProductName=PACCAR Technical Center MBDS Library
      settings: AttributesFormatString=|
      | Value: 8
      | Unit: '1'
  Constant4 : PTC_MBDS_LIB/Extras/Sources/Constant  Value2=GLB_TRAILER_TREAD_APV  PTC_MBDS_BlockVersion=5.41  PTC_BlockType=PTC_MBDS_Constant
      settings: SourceProductName=PACCAR Technical Center MBDS Library
      settings: AttributesFormatString=|
      | Value: 24
      | Unit: 'in/32'
  Constant5 : PTC_MBDS_LIB/Extras/Sources/Constant  Value2=GLB_NUMBER_OF_TRAILER_TIRES_APV  PTC_MBDS_BlockVersion=5.41  PTC_BlockType=PTC_MBDS_Constant
      settings: SourceProductName=PACCAR Technical Center MBDS Library
      settings: AttributesFormatString=|
      | Value: 8
      | Unit: '1'
  Divide : Product  Inputs=*/
  Divide1 : Product  Inputs=*/
  Divide2 : Product  Inputs=*/
  Gain : Gain  Gain=3
  Lookup Table1 : Lookup  InputValues=[-5:5]  Table=tanh([-5:5])  LookUpMeth=Interpolation-Use End Values
  Product : Product  Inputs=3  RndMeth=Zero
  Product1 : Product  Inputs=3  RndMeth=Zero
  Product2 : Product  Inputs=3  RndMeth=Zero
  Product5 : Product  RndMeth=Zero
  Unit Delay1 : UnitDelay  SampleTime=-1
  Unit Delay2 : UnitDelay  SampleTime=-1
  Unit Delay3 : UnitDelay  SampleTime=-1
  "Axle Forces X (N) " : Outport
  wires:
  Unit Delay2/1 -> 2D_Lookup_Table1/2
  Constant2/1 -> 2D_Lookup_Table1/1  "GLB_DRIVE_TREAD_APV"
  Constant1/1 -> Product/3, Divide/2  "GLB_NUMBER_OF_FRONT_TIRES_APV"
  Constant/1 -> 2D_Lookup_Table/1  "GLB_STEER_TREAD_APV"
  Constant5/1 -> Divide2/2, Product2/3  "GLB_NUMBER_OF_TRAILER_TIRES_APV"
  Divide2/1 -> Unit Delay3/1
  Constant3/1 -> Divide1/2, Product1/3  "GLB_NUMBER_OF_REAR_TIRES_APV"
  Divide1/1 -> Unit Delay2/1
  Divide/1 -> Unit Delay1/1
  Trailer Axle Load N/1 -> Divide2/1
  Constant4/1 -> 2D_Lookup_Table2/1  "GLB_TRAILER_TREAD_APV"
  Unit Delay3/1 -> 2D_Lookup_Table2/2
  Unit Delay1/1 -> 2D_Lookup_Table/2
  Drive Axle Load N/1 -> Divide1/1
  Front Axle Load N/1 -> Divide/1
  Product1/1 -> [RearTireLossForce], Bus Creator/2  "Rear Axle Force X (N)"
  2D_Lookup_Table/1 -> Product/2
  2D_Lookup_Table1/1 -> Product1/2
  Bus Creator/1 -> "Axle Forces X (N) "/1
  Gain/1 -> Lookup Table1/1
  Lookup Table1/1 -> [hyst]
  2D_Lookup_Table2/1 -> Product2/2
  [hyst] -> Product2/1
  Product/1 -> [FrontTireLossForce], Bus Creator/1  "Front Axle Force X"
  Product2/1 -> Bus Creator/3, [TrailerTireLossForce]  "Trailer Axle Force"
  Add4/1 -> Bus Creator/4, Product5/1  "Total Axle LossForce X"
  VehSpd(m/s)/1 -> Gain/1, Product5/2
  [FrontTireLossForce] -> Add4/1
  [RearTireLossForce] -> Add4/2
  [TrailerTireLossForce] -> Add4/3
  [hyst] -> Product/1
  [hyst] -> Product1/1
  Product5/1 -> Bus Creator/5  "TireResistancePower"

== system L4_SIM/Plant/PlantModel/Chassis/Chassis_SL/Chassis/Tractor lateral Model ==
  Steer Angle : Inport
  Vx : Inport  Port=2
  Fxf : Inport  Port=3
  VehMass : Inport  Port=4
  Abs : Abs
  Add : Sum  Inputs=+-+
  Add1 : Sum
  Add2 : Sum  Inputs=-+
  Add3 : Sum  Inputs=+-
  Add4 : Sum  Inputs=++-
  Add5 : Sum  Inputs=+-
  Cf : Constant  Value=Cf
  Compare To Constant : simulink/Logic and Bit Operations/Compare To Constant  relop=<=  const=0.01  OutDataTypeStr=boolean
  Cr : Constant  Value=Cr
  Divide : Product  Inputs=*/
  Divide1 : Product  Inputs=*/
  Fx_in : Scope
  Fy : Scope  NumInputPorts=2
  Gain : Gain  Gain=-1
  Gain1 : Gain  Gain=-1
  Inertia : Constant  Value=Iz
  Integrator : Integrator
  Integrator1 : Integrator
  Product{,1..8} (9 alike) : Product
  Product9 : Product  Inputs=3
  Slip : Scope  NumInputPorts=2
  Switch : Switch  Criteria=u2 > Threshold
  Trigonometric Function : Trigonometry  Operator=cos
  Trigonometric Function2 : Trigonometry
  Trigonometric Function3 : Trigonometry  Operator=atan2
  Trigonometric Function4 : Trigonometry  Operator=atan2
  Vx_in : Scope
  Vy&Yaw rate : Scope  NumInputPorts=2
  lf : Constant  Value=lf
  lr : Constant  Value=lr
  minVel : Constant  Value=0.01
  r : Scope  NumInputPorts=2
  Vy : Outport
  YawRate : Outport  Port=2
  wires:
  Product4/1 -> Add5/2  "Coriolis Force"
  Divide/1 -> Add5/1
  Add5/1 -> Integrator/1
  Trigonometric Function3/1 -> Add2/2
  Trigonometric Function4/1 -> Product1/1, Slip/2
  Add2/1 -> Product/2, Slip/1
  Trigonometric Function/1 -> Product3/1
  Product2/1 -> Add3/2
  Add1/1 -> Trigonometric Function3/1
  Product1/1 -> Gain1/1
  Add/1 -> Divide/1
  Product7/1 -> Add4/3
  Steer Angle/1 -> Trigonometric Function2/1, Trigonometric Function/1, Add2/1
  Add3/1 -> Trigonometric Function4/1
  Product5/1 -> Add1/1
  Divide1/1 -> Integrator1/1, r/1
  Cf/1 -> Product/1
  lf/1 -> Product5/1, Product6/1
  Product/1 -> Gain/1
  Cr/1 -> Product1/2
  Inertia/1 -> Divide1/2
  Fxf/1 -> Fx_in/1, Product8/1, Product9/2
  [lr] -> Product7/1, Product9/3
  Product9/1 -> Add4/1
  Integrator/1 -> Add3/1, Add1/2, Vy/1, Vy&Yaw rate/1  "Vy"
  Product3/1 -> Add/1, Product6/2
  Gain/1 -> Fy/1, Product3/2  "Fyf"
  Gain1/1 -> Fy/2, Product7/2, Add/3  "Fyr"
  Add4/1 -> Divide1/1
  Vx/1 -> Vx_in/1, Switch/3, Abs/1
  Product8/1 -> Add/2
  Product6/1 -> Add4/2
  Integrator1/1 -> Vy&Yaw rate/2, YawRate/1, r/2, Product2/1, Product5/2, Product4/2  "Yaw Rate"
  lr/1 -> Product2/2, [lr]
  Trigonometric Function2/1 -> Product8/2, Product9/1
  VehMass/1 -> Divide/2
  Abs/1 -> Compare To Constant/1
  Compare To Constant/1 -> Switch/2
  Switch/1 -> Trigonometric Function4/2, Trigonometric Function3/2, Product4/1
  minVel/1 -> Switch/1

== system L4_SIM/Plant/PlantModel/Chassis/Chassis_SL/Chassis/Trailer Model ==
  Vx : Inport
  heading : Inport  Port=2
  Divide : Product  Inputs=**/
  IC : InitialCondition  Value=0
  Sum2 : Sum  Inputs=|+-
  Trailer Heading : Integrator  InitialCondition=heading_0  UpperSaturationLimit=pi  LowerSaturationLimit=-pi  WrapState=on  WrappedStateUpperValue=2*pi  WrappedStateLowerValue=0
  Trailer Length : Constant  Value=15
  Trigonometric Function : Trigonometry
  wrap to pi1 : MATLAB Function  TreatAsAtomicUnit=on
  hitch angle : Outport
  wires:
  IC/1 -> hitch angle/1
  Vx/1 -> Divide/2
  wrap to pi1/1(y) -> Trigonometric Function/1, IC/1  "hitch angle"
  Divide/1 -> Trailer Heading/1
  Trailer Heading/1 -> Sum2/2
  Trailer Length/1 -> Divide/3
  heading/1 -> Sum2/1
  Sum2/1 -> wrap to pi1/1(u)
  Trigonometric Function/1 -> Divide/1

== system L4_SIM/Plant/PlantModel/Chassis/Chassis_SL/Chassis/Vehicle Dynamics ==
  beta : Inport
  Rho : Inport  Port=2
  Cd : Inport  Port=3
  Af : Inport  Port=4
  Mass : Inport  Port=5
  xDot : Inport  Port=6
  Aero : Subsystem
  Bus Creator : BusCreator  Inputs=2
  Constant : PTC_MBDS_LIB/Extras/Sources/Constant  Value2=GLB_GRAVITATIONAL_ACCELERATION_APV  PTC_MBDS_BlockVersion=5.41  PTC_BlockType=PTC_MBDS_Constant
      settings: SourceProductName=PACCAR Technical Center MBDS Library
      settings: AttributesFormatString=|
      | Value: 9.80665016174
      | Unit: 'm/s^2'
  Product1 : Product  Inputs=3  RndMeth=Zero
  Trigonometric Function : Trigonometry
  Dynamics : Outport
  AeroDragForce : Outport  Port=2
  InclineForce : Outport  Port=3
  wires:
  Constant/1 -> Product1/3  "GLB_GRAVITATIONAL_ACCELERATION_APV"
  xDot/1 -> Aero/4(xDot)
  Aero/1(AeroDragForce) -> Bus Creator/1, AeroDragForce/1  "AeroDragForce"
  Af/1 -> Aero/3(Af)
  Cd/1 -> Aero/2(Cd)
  Rho/1 -> Aero/1(Rho)
  Trigonometric Function/1 -> Product1/2
  Mass/1 -> Product1/1
  Product1/1 -> InclineForce/1, Bus Creator/2  "InclineForce"
  beta/1 -> Trigonometric Function/1
  Bus Creator/1 -> Dynamics/1

== system L4_SIM/Plant/PlantModel/Chassis/Chassis_SL/DriveAxleLosses/Divide_gtz ==
  num : Inport
  den : Inport  Port=2
  Enable : EnablePort
  Divide : Product  Inputs=*/
  out : Outport  OutputWhenDisabled=reset  InitialOutput=0
  wires:
  den/1 -> Divide/2
  num/1 -> Divide/1
  Divide/1 -> out/1

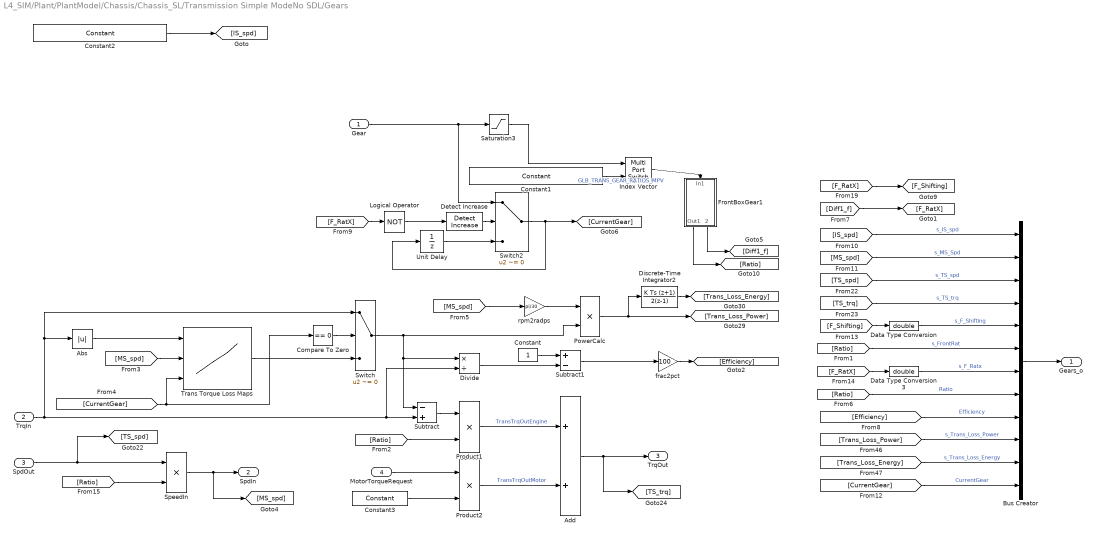
== system L4_SIM/Plant/PlantModel/Chassis/Chassis_SL/Transmission Simple ModeNo SDL/Gears ==
  Gear : Inport
  TrqIn : Inport  Port=2
  SpdOut : Inport  Port=3
  MotorTorqueRequest : Inport  Port=4
  Abs : Abs
  Add : Sum
  Bus Creator : BusCreator  Inputs=12
  Compare To Zero : simulink/Logic and Bit Operations/Compare To Zero  relop===  OutDataTypeStr=boolean
  Constant : Constant
  Constant1 : PTC_MBDS_LIB/Extras/Sources/Constant  Value2=GLB_TRANS_GEAR_RATIOS_MPV  PTC_MBDS_BlockVersion=5.41  PTC_BlockType=PTC_MBDS_Constant
      settings: SourceProductName=PACCAR Technical Center MBDS Library
      settings: AttributesFormatString=|
      | Value: <1 X 12>
      | Unit: '1'
  Constant2 : PTC_MBDS_LIB/Extras/Sources/Constant  Value2=0  PTC_MBDS_BlockVersion=5.41  PTC_BlockType=PTC_MBDS_Constant
      settings: SourceProductName=PACCAR Technical Center MBDS Library
  Constant3 : PTC_MBDS_LIB/Extras/Sources/Constant  Value2=1  PTC_MBDS_BlockVersion=5.41  PTC_BlockType=PTC_MBDS_Constant
      settings: SourceProductName=PACCAR Technical Center MBDS Library
  Data Type Conversion : DataTypeConversion  OutDataTypeStr=double
  Data Type Conversion3 : DataTypeConversion  OutDataTypeStr=double
  Detect Increase : simulink/Logic and Bit Operations/Detect Increase  vinit=0.0  OutDataTypeStr=boolean
  Discrete-Time Integrator2 : DiscreteIntegrator  IntegratorMethod=Integration: Trapezoidal  SampleTime=GLB_FIXED_STEP_SIZE_CPV  ICPrevOutput=DiscIntNeverNeededParam  ICPrevScaledInput=DiscIntNeverNeededParam
  Divide : Product  Inputs=*/
  FrontBoxGear1 : Subsystem
  Index Vector : MultiPortSwitch  Inputs=1
  Logical Operator : Logic  Operator=NOT  AllPortsSameDT=off  OutDataTypeStr=boolean
  PowerCalc : Product
  Product1 : Product
  Product2 : Product
  Saturation3 : Saturate  UpperLimit=inf  LowerLimit=1
  SpeedIn : Product
  Subtract : Sum  Inputs=-+
  Subtract1 : Sum  Inputs=+-
  Switch : Switch  Criteria=u2 ~= 0
  Switch2 : Switch  Criteria=u2 ~= 0
  Trans Torque Loss Maps : Lookup_n-D  NumberOfTableDimensions=3  BreakpointsForDimension1=GLB_TRANS_LOSS_TRQ_TRQ_STEP_MPV  BreakpointsForDimension2=GLB_TRANS_LOSS_TRQ_SPD_STEP_MPV  BreakpointsForDimension3=GLB_TRANS_LOSS_TRQ_GEAR_STEP_MPV  BeginIndexSearchUsingPreviousIndexResult=on  Table=GLB_TRANS_LOSS_TRQ_TABLE_DATA_MPV  InternalRulePriority=Speed  RndMeth=Simplest  InputSameDT=on
  Unit Delay : UnitDelay  SampleTime=-1
  frac2pct : Gain  Gain=100
  rpm2radps : Gain  Gain=pi/30
  Gears_o : Outport
  SpdIn : Outport  Port=2
  TrqOut : Outport  Port=3
  wires:
  Constant2/1 -> [IS_spd]
  Subtract/1 -> Product1/1
  Divide/1 -> Subtract1/2
  Constant/1 -> Subtract1/1
  TrqIn/1 -> Abs/1, Switch/1, Divide/2, Subtract/2
  [Ratio] -> Bus Creator/8  "Ratio"
  Compare To Zero/1 -> Switch/2
  Trans Torque Loss Maps/1 -> Switch/3
  Abs/1 -> Trans Torque Loss Maps/1
  [CurrentGear] -> Compare To Zero/1, Trans Torque Loss Maps/3
  frac2pct/1 -> [Efficiency]
  Subtract1/1 -> frac2pct/1
  rpm2radps/1 -> PowerCalc/1
  [MS_spd] -> rpm2radps/1
  Switch/1 -> Subtract/1, Divide/1, PowerCalc/2
  [MS_spd] -> Trans Torque Loss Maps/2
  Saturation3/1 -> Index Vector/1
  Add/1 -> [TS_trq], TrqOut/1
  SpeedIn/1 -> SpdIn/1, [MS_spd]
  [Ratio] -> SpeedIn/2
  [Ratio] -> Product1/2
  [CurrentGear] -> Bus Creator/12  "CurrentGear"
  Detect Increase/1 -> Switch2/2
  Switch2/1 -> Unit Delay/1, [CurrentGear]
  [F_RatX] -> Logical Operator/1
  Logical Operator/1 -> Detect Increase/1
  Unit Delay/1 -> Switch2/3
  Bus Creator/1 -> Gears_o/1
  [F_Shifting] -> Data Type Conversion/1
  [TS_trq] -> Bus Creator/4  "s_TS_trq"
  [TS_spd] -> Bus Creator/3  "s_TS_spd"
  [MS_spd] -> Bus Creator/2  "s_MS_Spd"
  [IS_spd] -> Bus Creator/1  "s_IS_spd"
  Index Vector/1 -> FrontBoxGear1/1(In1)
  Gear/1 -> Saturation3/1, Switch2/1
  [F_RatX] -> Data Type Conversion3/1
  [F_RatX] -> [F_Shifting]
  FrontBoxGear1/1(Out1) -> [Ratio]
  FrontBoxGear1/2(Diff_F) -> [Diff1_f]
  SpdOut/1 -> SpeedIn/1, [TS_spd]
  [Diff1_f] -> [F_RatX]
  PowerCalc/1 -> Discrete-Time Integrator2/1, [Trans_Loss_Power]
  Discrete-Time Integrator2/1 -> [Trans_Loss_Energy]
  Constant1/1 -> Index Vector/2  "GLB_TRANS_GEAR_RATIOS_MPV"
  Data Type Conversion/1 -> Bus Creator/5  "s_F_Shifting"
  [Ratio] -> Bus Creator/6  "s_FrontRat"
  Data Type Conversion3/1 -> Bus Creator/7  "s_F_Ratx"
  [Efficiency] -> Bus Creator/9  "Efficiency"
  [Trans_Loss_Power] -> Bus Creator/10  "s_Trans_Loss_Power"
  [Trans_Loss_Energy] -> Bus Creator/11  "s_Trans_Loss_Energy"
  MotorTorqueRequest/1 -> Product2/1
  Product1/1 -> Add/1  "TransTrqOutEngine"
  Product2/1 -> Add/2  "TransTrqOutMotor"
  Constant3/1 -> Product2/2
